simulink model "EKF_slam_fused"  (R2021a)
settings: Solver=VariableStepAuto  StartTime=0.0  StopTime=P.SimTime  RelTol=1e-3
undefined symbols (not defined in the file or in its folder): drawvehiclef4, Estimator_SLAMLf1, Estimator_SLAMLf2, Estimator_SLAMLf3, fusion_filter, P, Sensor_model_v4
settings Model: Creator=sankepaa

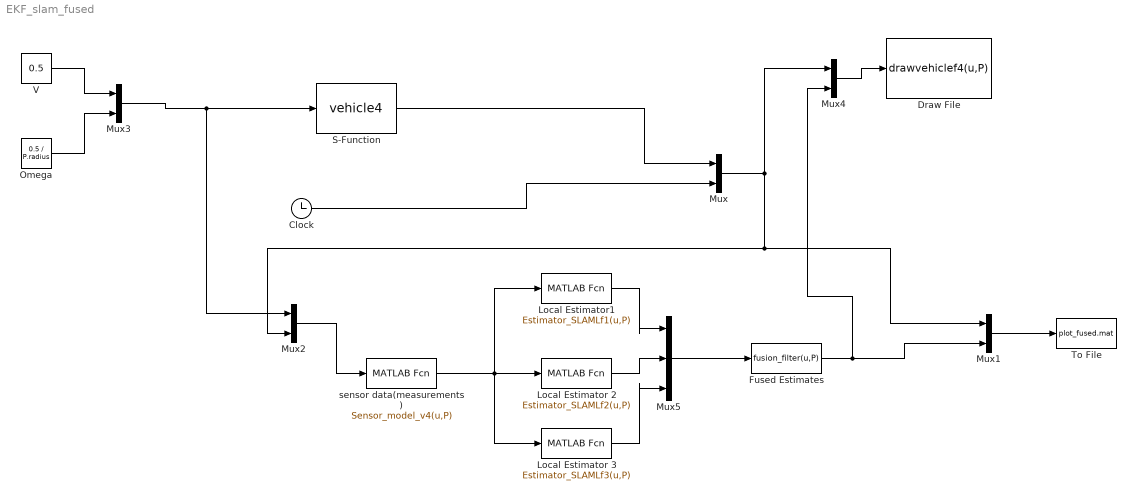
== system EKF_slam_fused ==
  " sensor data(measurements) " : MATLABFcn  MATLABFcn=Sensor_model_v4(u,P)  OutputDimensions=3*P.NumLm + 2 + 1
  Clock : Clock
  "Draw File " : MATLABFcn  MATLABFcn=drawvehiclef4(u,P)  OutputDimensions=0
  Fused Estimates : MATLABFcn  MATLABFcn=fusion_filter(u,P)  OutputDimensions=2*(3+2*P.NumLm)
  Local Estimator 2 : MATLABFcn  MATLABFcn=Estimator_SLAMLf2(u,P)  OutputDimensions=10
  Local Estimator 3 : MATLABFcn  MATLABFcn=Estimator_SLAMLf3(u,P)  OutputDimensions=10
  "Local Estimator1 " : MATLABFcn  MATLABFcn=Estimator_SLAMLf1(u,P)  OutputDimensions=10
  Mux{,1..4} (5 alike) : Mux  Inputs=2
  Mux5 : Mux  Inputs=3
  Omega : Constant  Value=0.5 / P.radius
  S-Function : S-Function  FunctionName=vehicle4  Parameters=P  SFunctionDeploymentMode=off  EnableBusSupport=off
  To File : ToFile  Filename=plot_fused.mat  MatrixName=dat  SaveFormat=Timeseries
  V : Constant  Value=0.5
  wires:
  S-Function/1 -> Mux/1
  Clock/1 -> Mux/2
  Mux/1 -> Mux4/1, Mux2/2, Mux1/1
  V/1 -> Mux3/1
  Omega/1 -> Mux3/2
  Mux3/1 -> Mux2/1, S-Function/1
  Mux2/1 -> " sensor data(measurements) "/1
  Mux4/1 -> "Draw File "/1
  " sensor data(measurements) "/1 -> Local Estimator 2/1, Local Estimator 3/1, "Local Estimator1 "/1
  "Local Estimator1 "/1 -> Mux5/1
  Local Estimator 2/1 -> Mux5/2
  Local Estimator 3/1 -> Mux5/3
  Mux5/1 -> Fused Estimates/1
  Fused Estimates/1 -> Mux4/2, Mux1/2
  Mux1/1 -> To File/1
